simulink library "SensorEx_Lib"  (Simulink 7.6)
settings: Solver=ode45  StartTime=0.0  StopTime=10.0  RelTol=1e-3
libraries: realtime_pacer_lib x2
settings Model: Creator=Tarex  LastModifiedBy=Tarex

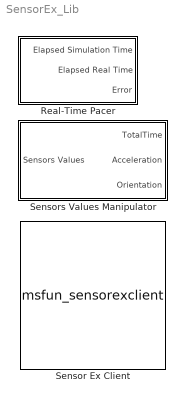
== system SensorEx_Lib ==
  Real-Time Pacer : Subsystem
      mask Type: Real-Time Pacer
      mask Description:
      | Derived from RealTime_Pacer can be found on the web.
      | 
      | Slow down a simulation to track real (i.e., wall clock) elapsed time.
      | 
      | Click on the Help button for details.
      mask Help: web('realtime_pacer_help.html', '-helpbrowser')
  Sensor Ex Client : M-S-Function  FunctionName=msfun_sensorexclient  Parameters=deviceNumber, imgSize  mask(Sensor Ex Client){deviceNumber=1, imgSize=[640 480]}
      mask prompts: deviceNumber "Device Number"; imgSize "Maximum Image Size [ImageHeight ImageWidth]"
      mask help: Matlab client for Sensor Ex application.
      mask Help: web('sensorexclient_help.html', '-helpbrowser')
      mask StyleString: popup(1|2|3|4|5),edit
      mask Display:
      | image(imread('sensorex.png','BackGroundColor',[1 0.5 0]), 'center')
      | 
      | port_label('output', 1, 'IP Local')
      | port_label('output', 2, 'IP Device')
      | port_label('output', 3, 'Sensors')
      | port_label('output', 4, 'R')
      | port_label('output', 5, 'G')
      | port_label('output', 6, 'B')
      | port_label('output', 7, 'FPS')
  Sensors Values Manipulator : Subsystem  mask(Sensors){outType=Standard, outStampT=off}
      mask prompts: outType "Output Type"; outStampT "Output Time Stamp"
      mask help: Manipulate sensors values fed by a Sensor Ex Client.
      mask init:
      | refblock = [gcb '/Sensors Values'];
      | posRef = get_param(refblock,'Position');
      | 
      | inioffsetX = 300;
      | sizInport = [30 15];
      | sizDemux = [10 200];
      | sizMux = [10 100];
      | 
      | posReff = [posRef(1)+inioffsetX (posRef(4)+posRef(2))/2];
      | % pos = [365   103   395   117];
      | % pos = [posReff(1) posReff(2)-siz(2)/2 posReff(1)+siz(1) posReff(2)+siz(2)/2];
      | pos = [posReff(1) posReff(2) posReff(1) posReff(2)];
      | 
      | switch outType
      |     case 'Standard'    
      |         try
      |             delete_line(gcb,'Demux/3','AccX/1')
      |             delete_line(gcb,'Demux/4','AccY/1')
      |             delete_line(gcb,'Demux/5','AccZ/1')
      |             
      |             delete_line(gcb,'Demux/6','OriX/1')
      |             delete_line(gcb,'Demux/7','OriY/1')
      |             delete_line(gcb,'Demux/8','OriZ/1')
      |             
      |             
      |             delete_block([gcb '/AccX']);
      |             delete_block([gcb '/AccY']);
      |             delete_block([gcb '/AccZ']);
      |             
      |             delete_block([gcb '/OriX']);
      |             delete_block([gcb '/OriY']);
      |             delete_block([gcb '/OriZ']);
      |             
      |             %             delete_unconnected_lines(gcb);
      |             
      |             add_blk('built-in/Outport',[gcb '/Acceleration'],pos,[0,-15],sizInport);
      |             add_blk('built-in/Outport',[gcb '/Orientation'],pos,[0,90],sizInport);
      |             %         add_blk('built-in/Outport',[gcb '/TimeStamp'],pos,[0,100],sizInport);
      |             
      |             %         add_blk('built-in/Demux',[gcb '/Demux'],pos,[-inioffsetX*2/3,0],sizDemux);
      |             %         set_param([gcb '/Demux'],'Outputs','7','DisplayOption','bar');
      |             
      |             add_blk('built-in/Mux',[gcb '/MuxAcc'],pos,[-inioffsetX/3,-25],sizMux);
      |             set_param([gcb '/MuxAcc'],'Inputs','3','DisplayOption','bar');
      |             
      |             add_blk('built-in/Mux',[gcb '/MuxOri'],pos,[-inioffsetX/3,80],sizMux);
      |             set_param([gcb '/MuxOri'],'Inputs','3','DisplayOption','bar');
      |             
      |             %         add_line(gcb,'Fetch Sensors Values/1','Demux/1','autorouting','on')
      |             
      |             add_line(gcb,'Demux/3','MuxAcc/1','autorouting','on')
      |             add_line(gcb,'Demux/4','MuxAcc/2','autorouting','on')
      |             add_line(gcb,'Demux/5','MuxAcc/3','autorouting','on')
      |             add_line(gcb,'MuxAcc/1','Acceleration/1','autorouting','on')
      |             
      |             add_line(gcb,'Demux/6','MuxOri/1','autorouting','on')
      |             add_line(gcb,'Demux/7','MuxOri/2','autorouting','on')
      |             add_line(gcb,'Demux/8','MuxOri/3','autorouting','on')
      |             add_line(gcb,'MuxOri/1','Orientation/1','autorouting','on')
      |             
      |             %         add_line(gcb,'Demux/7','TimeStamp/1','autorouting','on')
      |             
      |             %     case 'Single Array'
      |             %
      |             %         add_blk('built-in/Outport',[gcb '/Values'],pos,[0,0],sizInport);
      |             %
      |             %         add_line(gcb,'Fetch Sensors Values/1','Values/1','autorouting','on')
      |             
      |         end
      |     case 'Divided Arrays'      
      |         try
      |             delete_line(gcb,'Demux/3','MuxAcc/1')
      |             delete_line(gcb,'Demux/4','MuxAcc/2')
      |             delete_line(gcb,'Demux/5','MuxAcc/3')
      |             delete_line(gcb,'MuxAcc/1','Acceleration/1')
      |             
      |             delete_line(gcb,'Demux/6','MuxOri/1')
      |             delete_line(gcb,'Demux/7','MuxOri/2')
      |             delete_line(gcb,'Demux/8','MuxOri/3')
      |             delete_line(gcb,'MuxOri/1','Orientation/1')
      |             
      |             
      |             delete_block([gcb '/Acceleration']);
      |             delete_block([gcb '/Orientation']);
      |             
      |             delete_block([gcb '/MuxAcc']);
      |             delete_block([gcb '/MuxOri']);
      |             
      |             %             delete_unconnected_lines(gcb);
      |             
      |             dist = 20;
      |             
      |             add_blk('built-in/Outport',[gcb '/AccX'],pos,[0,-3*(dist-2)],sizInport);
      |             add_blk('built-in/Outport',[gcb '/AccY'],pos,[0,-1*dist],sizInport);
      |             add_blk('built-in/Outport',[gcb '/AccZ'],pos,[0,1*(dist-5)],sizInport);
      |             
      |             add_blk('built-in/Outport',[gcb '/OriX'],pos,[0,3*(dist-3)],sizInport);
      |             add_blk('built-in/Outport',[gcb '/OriY'],pos,[0,5*(dist-3)],sizInport);
      |             add_blk('built-in/Outport',[gcb '/OriZ'],pos,[0,8*(dist-5)],sizInport);
      |             
      |             %         add_blk('built-in/Demux',[gcb '/Demux'],pos,[-inioffsetX/2,0],sizDemux);
      |             %         set_param([gcb '/Demux'],'Outputs','7','DisplayOption','bar');
      |             
      |             %         add_line(gcb,'Fetch Sensors Values/1','Demux/1','autorouting','on')
      |             
      |             add_line(gcb,'Demux/3','AccX/1','autorouting','on')
      |             add_line(gcb,'Demux/4','AccY/1','autorouting','on')
      |             add_line(gcb,'Demux/5','AccZ/1','autorouting','on')
      |             
      |             add_line(gcb,'Demux/6','OriX/1','autorouting','on')
      |             add_line(gcb,'Demux/7','OriY/1','autorouting','on')
      |             add_line(gcb,'Demux/8','OriZ/1','autorouting','on')        
      |         end       
      | end
      | 
      | if strcmp(outStampT,'on')
      |     try
      |         delete_line(gcb,'Demux/2','Terminator/1')
      |         
      |         delete_block([gcb '/Terminator']);
      |         
      |         add_blk('built-in/Outport',[gcb '/TimeStamp'],pos,[0,-90],sizInport);
      |         add_line(gcb,'Demux/2','TimeStamp/1','autorouting','on')
      |         set_param([gcb '/TimeStamp'],'Port',num2str(2))
      |     end
      | else
      |     try
      |         delete_line(gcb,'Demux/2','TimeStamp/1')
      |         
      |         delete_block([gcb '/TimeStamp']);
      |         
      |         add_blk('built-in/Terminator',[gcb '/Terminator'],pos,[0,-90],sizInport);
      |         add_line(gcb,'Demux/2','Terminator/1','autorouting','on')
      |     end
      | end
      | 
      | % color('red'); port_label('output',1,'Varun')
      | 
      | % if strcmp(outTotalT,'on')
      | %     add_blk('built-in/Outport',[gcb '/TotalTime'],pos,[0,133],sizInport);
      | %     add_line(gcb,'Demux/7','TotalTime/1','autorouting','on')
      | % else
      | %
      | % end
      | 
      | % n = 1;
      | % if strcmp(outType,'Divided Arrays')
      | %     set_param([gcb '/Values'],'Port',num2str(n))
      | %     n = 2; % increase n
      | % end
      mask Help: web('sensorsvaluesmanipulator_help.html', '-helpbrowser')
      mask StyleString: popup(Standard|Divided Arrays),checkbox
      mask Display:
      | % image(imread('sensorex_graph.png'))
      | % color('red'); port_label('output',1,'Varun')
      | % patch([0 10 20 30 30 0], [10 30 20 25 10 10],[1 0 0])

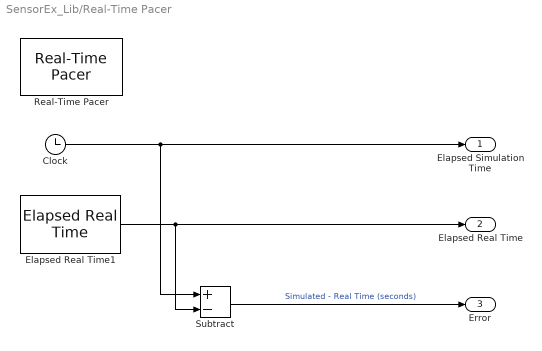
== system SensorEx_Lib/Real-Time Pacer ==
  Clock : Clock
      settings: Decimation=10
  Elapsed Real Time1 : realtime_pacer_lib/Elapsed Real Time
  Real-Time Pacer : realtime_pacer_lib/Real-Time Pacer  simTimePerRealTime=1
  Subtract : Sum  Inputs=+-
  Elapsed Simulation Time : Outport
  Elapsed Real Time : Outport  Port=2
  Error : Outport  Port=3
  wires:
  Clock/1 -> Subtract/1, Elapsed Simulation Time/1
  Subtract/1 -> Error/1  "Simulated - Real Time (seconds)"
  Elapsed Real Time1/1 -> Subtract/2, Elapsed Real Time/1

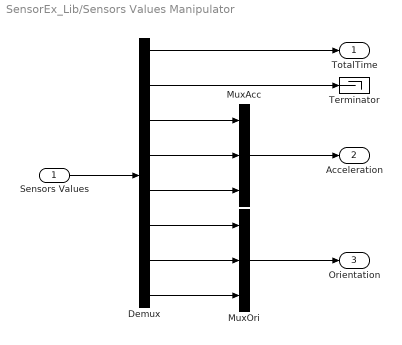
== system SensorEx_Lib/Sensors Values Manipulator ==
  Sensors Values : Inport
  Demux : Demux  Outputs=8
  MuxAcc : Mux  Inputs=3
  MuxOri : Mux  Inputs=3
  Terminator : Terminator
  TotalTime : Outport
  Acceleration : Outport  Port=2
  Orientation : Outport  Port=3
  wires:
  Sensors Values/1 -> Demux/1
  Demux/1 -> TotalTime/1
  Demux/3 -> MuxAcc/1
  Demux/4 -> MuxAcc/2
  Demux/5 -> MuxAcc/3
  MuxAcc/1 -> Acceleration/1
  Demux/6 -> MuxOri/1
  Demux/7 -> MuxOri/2
  Demux/8 -> MuxOri/3
  MuxOri/1 -> Orientation/1
  Demux/2 -> Terminator/1
